simulink model "Commander_Stabilizer_QDrone_Follower"  (Simulink 9.1)
settings: Solver=ode1  StartTime=0.0  StopTime=inf  FixedStep=0.001  RelTol=1e-3  EnableMultiTasking=on
model workspace (MAT data in the model file):
  target_system : num (value not decoded)
InitFcn:
  | set_param(gcs, 'ZoomFactor','FitSystem')
undefined symbols (not defined in the file): HIL, qc_get_step_size
libraries: quarc_library x62, simulink x24, simulink_extras x5
(part 1 of 4)
settings Model: Creator=dmadill  LastModifiedBy=jpineros  SimulationMode=external  ExtModeTrigDuration=10000
settings SolverCC: PositivePriorityOrder=on
settings DataIOCC: LimitDataPoints=on
settings OptimizationCC: LifeSpan=auto
settings DebuggingCC: UnderspecifiedInitializationDetection=Simplified  MergeDetectMultiDrivingBlocksExec=error  SolverPrmCheckMsg=warning
settings HardwareCC: ProdBitPerLong=64  ProdBitPerPointer=64  ProdBitPerSizeT=64  ProdBitPerPtrDiffT=64  ProdLargestAtomicFloat=Float  ProdIntDivRoundTo=Zero  ProdEndianess=LittleEndian  ProdWordSize=64  ProdHWDeviceType=Intel->x86-64 (Linux 64)
settings RTWCC: SystemTargetFile=quarc_linux_x64.tlc  TemplateMakefile=quarc_linux_x64_tmf  Description=QUARC Linux x64 Target (QDrone)  BuildConfiguration=Faster Runs
settings STFCustomTargetCC: TargetLibSuffix=.a  ConcurrentExecutionCompliant=on  SystemTargetFile=quarc_linux_x64.tlc
settings GRTTargetCC: TargetLibSuffix=.a  TargetPreCompLibLocation=C:\PROGRA~3\QUARC\lib\2018a\LIA7F9~1\release  ParMdlRefBuildCompliant=off  CompOptLevelCompliant=off  MatFileLogging=off  CPPClassGenCompliant=off  UseToolchainInfoCompliant=off  ExtMode=on  ExtModeMexFile=quarc_comm  ExtModeMexArgs='-w -d /tmp -uri %u'
settings ConfigComp: CovHtmlReporting=off  CovSFcnEnable=off

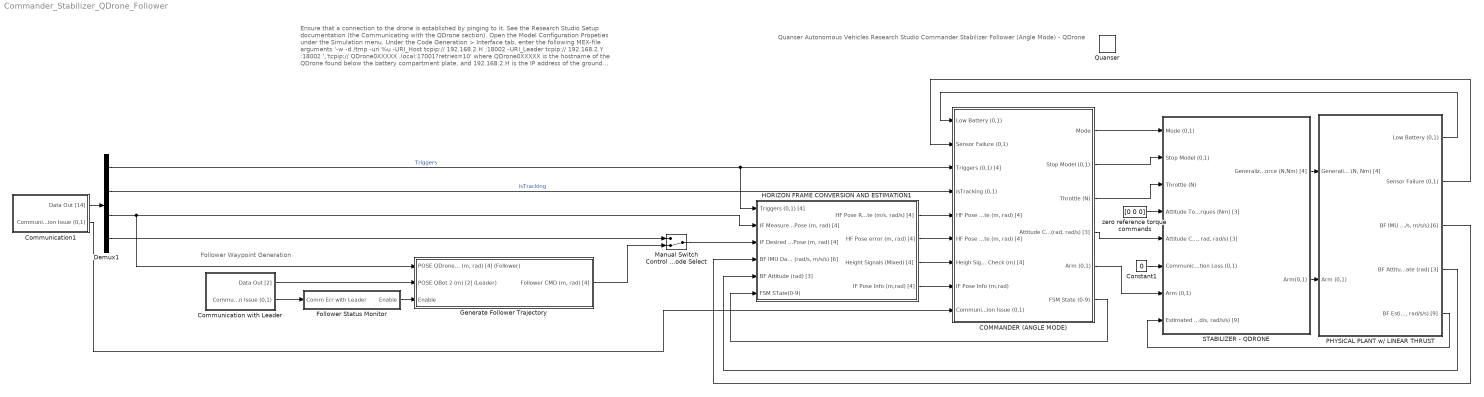
== system Commander_Stabilizer_QDrone_Follower ==
  note: Follower Waypoint Generation
  note: Quanser Autonomous Vehicles Research Studio
      | Commander Stabilizer Follower (Angle Mode) - QDrone
  note: Ensure that a connection to the drone is established by pinging to it. See the Research Studio Setup documentation (the Communicating with the QDrone section).
      | Open the Model Configuration Propeties under the Simulation menu.
      | Under the Code Generation > Interface tab, enter the following MEX-file arguments
      | '-w -d /tmp -uri %u -URI_Host tcpip:// 192.168.2.H :18002 -URI_Leader tcpip:// 192.168.2.Y :18002 ','tcpip:// QDrone0XXXXX .local:17001?retries=10'
      | where QDrone0XXXXX is the hostname of the QDrone found below the battery compartment plate, and 192.168.2.H is the IP address of the ground control station PC (should be 192.168.2.5 by default), 192.168.2.Y . is the IP address of the QBot2e which can be found on the custom Quanser PCB.
      |
      | Under the QUARC menu, click on Build .
      |
      | Ensure that the Mission Server Leader Follower model is running. If not, this model will stop immediately upon running. Click on Start under the QUARC menu.
      |
      | Ensure that the drone behaves as expected (see the steps in the Mission Server Leader Follower model)
      | This model will automatically stop when the QDrone lands.
  COMMANDER (ANGLE MODE) : Subsystem
  Communication with Leader : Subsystem
  Communication1 : Subsystem
  Constant1 : Constant  Value=0
  Demux1 : Demux  Outputs=[4 1 4 4]
  Follower Status Monitor : Subsystem
  Generate Follower Trajectory : Subsystem
  HORIZON FRAME CONVERSION AND ESTIMATION1 : Subsystem
  Manual Switch Control Mode Select : ManualSwitch  CurrentSetting=0
  PHYSICAL PLANT w/ LINEAR THRUST : Subsystem
  Quanser : quarc_library/Logos/Quanser
  STABILIZER - QDRONE : Subsystem
  zero reference torque commands : Constant  Value=[0 0 0]
  wires:
  Communication with Leader/1(Data Out [2]) -> Generate Follower Trajectory/2(POSE QBot 2 (m) [2] (Leader))
  Generate Follower Trajectory/1("Follower CMD (m, rad) [4]") -> Manual Switch Control Mode Select/2
  Follower Status Monitor/1(Enable) -> Generate Follower Trajectory/3(Enable)
  Communication with Leader/2(Communication Issue (0,1)) -> Follower Status Monitor/1(Comm Err with Leader)
  HORIZON FRAME CONVERSION AND ESTIMATION1/2("HF Pose error (m, rad) [4]") -> COMMANDER (ANGLE MODE)/6("HF Pose Error  Estimate (m, rad) [4]")
  HORIZON FRAME CONVERSION AND ESTIMATION1/1("HF Pose Rate  Estimate (m/s, rad/s) [4]") -> COMMANDER (ANGLE MODE)/5("HF Pose Rate  Estimate (m, rad) [4]")
  PHYSICAL PLANT w/ LINEAR THRUST/3("BF IMU Data (rad/s, m/s/s) [6]") -> HORIZON FRAME CONVERSION AND ESTIMATION1/4("BF IMU Data  (rad/s, m/s/s) [6]")
  COMMANDER (ANGLE MODE)/6(FSM State (0-9)) -> HORIZON FRAME CONVERSION AND ESTIMATION1/6(FSM STate(0-9))
  HORIZON FRAME CONVERSION AND ESTIMATION1/3(Height Signals (Mixed) [4]) -> COMMANDER (ANGLE MODE)/7(Heigh Signals Check (m) [4])
  Demux1/2 -> COMMANDER (ANGLE MODE)/4(isTracking (0,1))  "isTracking"
  Communication1/2(Communication Issue (0,1)) -> COMMANDER (ANGLE MODE)/9(Communication Issue (0,1))
  Demux1/3 -> Generate Follower Trajectory/1("POSE QDrone (m, rad) [4] (Follower)"), HORIZON FRAME CONVERSION AND ESTIMATION1/2("IF Measured Pose (m, rad) [4]")
  zero reference torque commands/1 -> STABILIZER - QDRONE/4(Attitude Torques (Nm) [3])
  COMMANDER (ANGLE MODE)/1(Mode) -> STABILIZER - QDRONE/1(Mode (0,1))
  COMMANDER (ANGLE MODE)/4("Attitude Commands (rad, rad/s) [3]") -> STABILIZER - QDRONE/5("Attitude Commands (rad, rad, rad/s) [3]")
  Demux1/1 -> COMMANDER (ANGLE MODE)/3(Triggers (0,1) [4]), HORIZON FRAME CONVERSION AND ESTIMATION1/1(Triggers (0,1) [4])  "Triggers"
  COMMANDER (ANGLE MODE)/3(Throttle (N)) -> STABILIZER - QDRONE/3(Throttle (N))
  Constant1/1 -> STABILIZER - QDRONE/6(Communication Loss (0,1))
  COMMANDER (ANGLE MODE)/5(Arm (0,1)) -> STABILIZER - QDRONE/7(Arm (0,1))
  Communication1/1(Data Out [14]) -> Demux1/1
  PHYSICAL PLANT w/ LINEAR THRUST/2(Sensor Failure (0,1)) -> COMMANDER (ANGLE MODE)/2(Sensor Failure (0,1))
  PHYSICAL PLANT w/ LINEAR THRUST/4(" BF Attitude Estimate (rad) [3]") -> HORIZON FRAME CONVERSION AND ESTIMATION1/5(BF Attitude (rad) [3])
  PHYSICAL PLANT w/ LINEAR THRUST/5("BF Estimated Attitude (rad, rad/s, rad/s/s) [9]") -> STABILIZER - QDRONE/8("Estimated Attitude (rad, rad/s, rad/s/s) [9]")
  STABILIZER - QDRONE/1(Generalized  Force (N,Nm) [4]) -> PHYSICAL PLANT w/ LINEAR THRUST/1("Generalized Force (N, Nm) [4]")
  STABILIZER - QDRONE/2(Arm(0,1)) -> PHYSICAL PLANT w/ LINEAR THRUST/2(Arm (0,1))
  COMMANDER (ANGLE MODE)/2(Stop Model (0,1)) -> STABILIZER - QDRONE/2(Stop Model (0,1))
  PHYSICAL PLANT w/ LINEAR THRUST/1(Low Battery (0,1)) -> COMMANDER (ANGLE MODE)/1(Low Battery (0,1))
  HORIZON FRAME CONVERSION AND ESTIMATION1/4(IF Pose Info (m,rad) [4]) -> COMMANDER (ANGLE MODE)/8(IF Pose Info (m,rad))
  Demux1/4 -> Manual Switch Control Mode Select/1
  Manual Switch Control Mode Select/1 -> HORIZON FRAME CONVERSION AND ESTIMATION1/3("IF Desired Pose (m, rad) [4]")

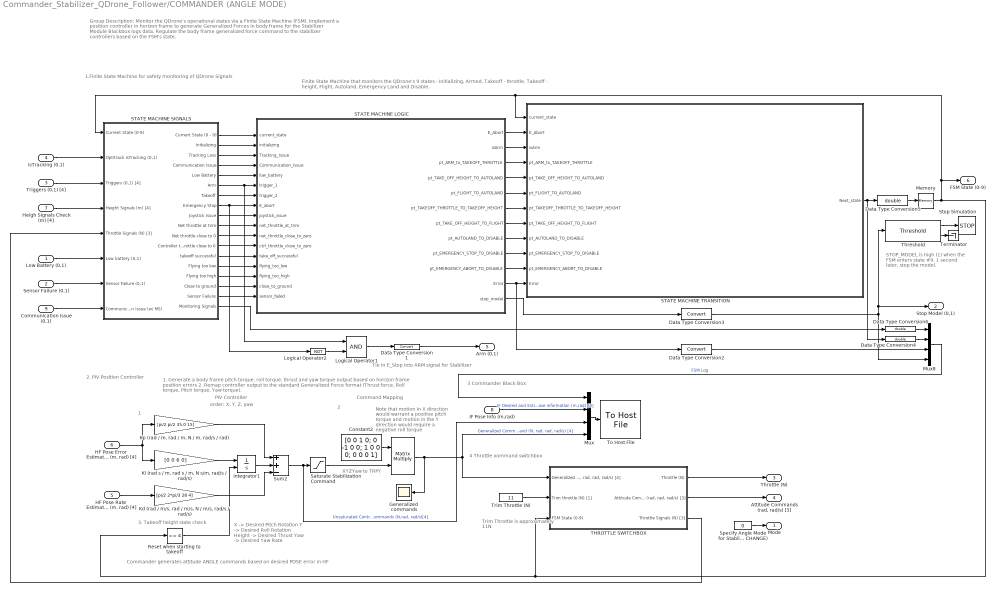
== system Commander_Stabilizer_QDrone_Follower/COMMANDER (ANGLE MODE) ==
  note: STOP_MODEL is high (1) when
      | the FSM enters state #9.
      | 1 second later, stop the model.
  note: Tie in E_Stop into ARM signal for Stabilizer
  note: Finite State Machine that monitors the QDrone's 9 states - Initializing, Armed, Takeoff - throttle, Takeoff - height, Flight, Autoland, Emergency Land and Disable.
  note: X -> Desired Pitch Rotation
      | Y -> Desired Roll Rotation
      | Height -> Desired Thrust
      | Yaw -> Desired Yaw Rate
  note: PIV Controller
  note: 2
  note: 1. Generate a body frame pitch torque, roll torque, thrust and yaw torque output based on horizon frame position errors
      | 2. Remap controller output to the standard Generalized Force format (Thrust force, Roll torque, Pitch torque, Yaw torque).
  note: order: X, Y, Z, yaw
  note: 3. Takeoff height state check
  note: 1
  note: XYZYaw to TRPY
  note: Command Mapping
  note: Note that motion in X direction would warrant a positive pitch torque
      | and motion in the Y direction would require a negative roll torque
  note: Trim Throttle is approximately 11N
  note: Group Description:
      |
      | Monitor the QDrone's operational states via a Finite State Machine (FSM).
      | Implement a position controller in horizon frame to generate Generalized Forces in body frame for the Stabilizer Module
      | Blackbox logs data.
      | Regulate the body frame generalized force command to the stabilizer controllers based on the FSM's state.
  note: 4 Throttle xommand switchbox
  note: 3 Commander Black Box
  note: Commander generates attitude ANGLE commands based on desired POSE error in HF
  note: 2. PIV Position Controller
  note: 1.Finite State Machine for safety monitoring of QDrone Signals
  Low Battery (0,1) : Inport
  Sensor Failure (0,1) : Inport  Port=2
  Triggers (0,1) [4] : Inport  Port=3
  isTracking (0,1) : Inport  Port=4
  "HF Pose Rate  Estimate (m, rad) [4]" : Inport  Port=5
  "HF Pose Error  Estimate (m, rad) [4]" : Inport  Port=6
  Heigh Signals Check (m) [4] : Inport  Port=7
  IF Pose Info (m,rad) : Inport  Port=8
  Communication Issue (0,1) : Inport  Port=9
  " " : Product  Multiplication=Matrix(*)
  Constant2 : Constant  Value=[0 0 1 0; 0 -1 0 0; 1 0 0 0; 0 0 0 1]
  Data Type Conversion1 : DataTypeConversion
  Data Type Conversion2 : DataTypeConversion
  Data Type Conversion3 : DataTypeConversion
  Data Type Conversion4 : DataTypeConversion  OutDataTypeStr=double
  Data Type Conversion5 : DataTypeConversion  OutDataTypeStr=double
  Data Type Conversion6 : DataTypeConversion  OutDataTypeStr=double
  "Generalized  commands " : Scope
  Integrator1 : Integrator  ExternalReset=rising  LimitOutput=on  UpperSaturationLimit=[0.26 0.33 15 0.05].*0.75  LowerSaturationLimit=[-0.26 -0.33 -15 -0.05].*0.75
  "Kd (rad / m/s, rad / m/s, N / m/s, rad/s / rad/s)" : Gain  Gain=[pi/2 2*pi/3 28 4]
  "Ki (rad s / m, rad s / m, N s/m, rad/s / rad/s)" : Gain  Gain=[0 0 6 0]
  "Kp (rad / m, rad / m, N / m, rad/s / rad)" : Gain  Gain=[pi/2 pi/2 35.0 15]
  Logical Operator1 : Logic  AllPortsSameDT=off  OutDataTypeStr=boolean
  Logical Operator2 : Logic  Operator=NOT  AllPortsSameDT=off  OutDataTypeStr=boolean
  Memory : Memory  InitialCondition=1
  Mux : Mux
  Mux8 : Mux  Inputs=[17 1 1 1]
  Reset when starting to takeoff : simulink/Logic and Bit Operations/Compare To Constant  relop===  const=4  OutDataTypeStr=boolean
  STATE MACHINE LOGIC : MATLAB Function  TreatAsAtomicUnit=on
  STATE MACHINE SIGNALS : Subsystem
  STATE MACHINE TRANSITION : MATLAB Function  TreatAsAtomicUnit=on
  Saturate Stabilization Command : Saturate  UpperLimit=[pi/4 pi/4 35 100*pi/180]  LowerLimit=[-pi/4 -pi/4 -35 -100*pi/180]
  Specify Angle Mode for Stabilizer (DO NOT CHANGE) : Constant  Value=0
  Stop Simulation : Stop
  Sum2 : Sum  Inputs=++-
  "THROTTLE SWITCHBOX " : Subsystem
  Terminator : Terminator
  Threshold : quarc_library/Discontinuities/Threshold  operator=>=  param_src=Specify via dialog  threshold=0.5  duration=1
      settings: SourceProductName=QUARC Targets
  To Host File : quarc_library/Sinks/To Host/To Host File  file_name=saved_data/%m/Commander_%{date}_%{time}.mat  variable_name=commander_data  decimation=1  sample_time=-1  file_format=MAT-file v.5  options=No header or footer  append=off  final_file_name=saved_data/Commander_Stabilizer_QDrone_Follower/Commander_20-Jan-2022_08-51-27.mat  bitrate=2000000
  "Trim Throttle (N) " : Constant  Value=11
  Mode : Outport
  Stop Model (0,1) : Outport  Port=2
  Throttle (N) : Outport  Port=3
  "Attitude Commands (rad, rad/s) [3]" : Outport  Port=4
  Arm (0,1) : Outport  Port=5
  FSM State (0-9) : Outport  Port=6
  wires:
  Heigh Signals Check (m) [4]/1 -> STATE MACHINE SIGNALS/4(Height Signals (m) [4])
  Triggers (0,1) [4]/1 -> STATE MACHINE SIGNALS/3(Triggers (0,1) [4])
  isTracking (0,1)/1 -> STATE MACHINE SIGNALS/2("Optitrack isTracking (0,1)  ")
  Communication Issue (0,1)/1 -> STATE MACHINE SIGNALS/8(Communication Issue (w/ MS))
  Sensor Failure (0,1)/1 -> STATE MACHINE SIGNALS/7(Sensor Failure (0,1))
  Low Battery (0,1)/1 -> STATE MACHINE SIGNALS/6(Low battery (0,1))
  STATE MACHINE LOGIC/11(Error) -> Data Type Conversion2/1, STATE MACHINE TRANSITION/12(Error)
  STATE MACHINE SIGNALS/17("  Sensor Failure") -> STATE MACHINE LOGIC/17(sensor_failed)
  STATE MACHINE LOGIC/8(pt_AUTOLAND_TO_DISABLE) -> STATE MACHINE TRANSITION/9(pt_AUTOLAND_TO_DISABLE)
  STATE MACHINE LOGIC/10(pt_EMERGENCY_ABORT_TO_DISABLE) -> STATE MACHINE TRANSITION/11(pt_EMERGENCY_ABORT_TO_DISABLE)
  Logical Operator2/1 -> Logical Operator1/2
  STATE MACHINE LOGIC/7(pt_TAKE_OFF_HEIGHT_TO_FLIGHT) -> STATE MACHINE TRANSITION/8(pt_TAKE_OFF_HEIGHT_TO_FLIGHT)
  STATE MACHINE SIGNALS/18(Monitoring Signals) -> Data Type Conversion6/1
  STATE MACHINE SIGNALS/6(Arm) -> STATE MACHINE LOGIC/6(trigger_1), Logical Operator1/1
  Logical Operator1/1 -> Data Type Conversion1/1
  Data Type Conversion2/1 -> Mux8/3
  Threshold/2 -> Terminator/1
  STATE MACHINE LOGIC/4(pt_TAKE_OFF_HEIGHT_TO_AUTOLAND) -> STATE MACHINE TRANSITION/5(pt_TAKE_OFF_HEIGHT_TO_AUTOLAND)
  Data Type Conversion3/1 -> Mux8/4, Threshold/1, Stop Model (0,1)/1
  STATE MACHINE LOGIC/2(isArm) -> STATE MACHINE TRANSITION/3(isArm)
  Data Type Conversion1/1 -> Arm (0,1)/1
  STATE MACHINE SIGNALS/2(Initializing) -> STATE MACHINE LOGIC/2(initializing)
  STATE MACHINE SIGNALS/3(Tracking Loss) -> STATE MACHINE LOGIC/3(Tracking_Issue)
  STATE MACHINE SIGNALS/10(Net throttle at trim) -> STATE MACHINE LOGIC/10(net_throttle_at_trim)
  STATE MACHINE SIGNALS/15(Flying too high) -> STATE MACHINE LOGIC/15(flying_too_high)
  STATE MACHINE SIGNALS/14(Flying too low) -> STATE MACHINE LOGIC/14(flying_too_low)
  STATE MACHINE SIGNALS/12(Controller throttle close to 0) -> STATE MACHINE LOGIC/12(ctrl_throttle_close_to_zero)
  Data Type Conversion4/1 -> Mux8/2
  STATE MACHINE SIGNALS/9("Joystick Issue ") -> STATE MACHINE LOGIC/9(joystick_issue)
  STATE MACHINE LOGIC/1(E_Abort) -> STATE MACHINE TRANSITION/2(E_Abort)
  STATE MACHINE LOGIC/5(pt_FLIGHT_TO_AUTOLAND) -> STATE MACHINE TRANSITION/6(pt_FLIGHT_TO_AUTOLAND)
  STATE MACHINE LOGIC/9(pt_EMERGENCY_STOP_TO_DISABLE) -> STATE MACHINE TRANSITION/10(pt_EMERGENCY_STOP_TO_DISABLE)
  STATE MACHINE SIGNALS/4(Communication Issue) -> STATE MACHINE LOGIC/4(Communication_Issue)
  STATE MACHINE TRANSITION/1(Next_state) -> Data Type Conversion4/1, Data Type Conversion5/1
  STATE MACHINE SIGNALS/7(Takeoff) -> STATE MACHINE LOGIC/7(trigger_2)
  STATE MACHINE SIGNALS/13(takeoff successful) -> STATE MACHINE LOGIC/13(take_off_successful)
  STATE MACHINE LOGIC/12(stop_model) -> Data Type Conversion3/1
  STATE MACHINE LOGIC/6(pt_TAKEOFF_THROTTLE_TO_TAKEOFF_HEIGHT) -> STATE MACHINE TRANSITION/7(pt_TAKEOFF_THROTTLE_TO_TAKEOFF_HEIGHT)
  STATE MACHINE SIGNALS/16(Close to ground) -> STATE MACHINE LOGIC/16(close_to_ground)
  STATE MACHINE SIGNALS/11(Net throttle close to 0) -> STATE MACHINE LOGIC/11(net_throttle_close_to_zero)
  Data Type Conversion6/1 -> Mux8/1
  STATE MACHINE SIGNALS/8(Emergency Stop) -> STATE MACHINE LOGIC/8(E_abort), Logical Operator2/1
  STATE MACHINE SIGNALS/5(Low Battery) -> STATE MACHINE LOGIC/5(low_battery)
  Data Type Conversion5/1 -> Memory/1
  STATE MACHINE LOGIC/3(pt_ARM_to_TAKEOFF_THROTTLE) -> STATE MACHINE TRANSITION/4(pt_ARM_to_TAKEOFF_THROTTLE)
  Threshold/1 -> Stop Simulation/1
  STATE MACHINE SIGNALS/1("Current State (0 - 9)  ") -> STATE MACHINE LOGIC/1(current_state)
  " "/1 -> Mux/4, "THROTTLE SWITCHBOX "/1("Generalized Command (N, rad, rad, rad/s) [4]"), "Generalized  commands "/1  "Generalized Command (N, rad, rad, rad/s) [4]"
  Reset when starting to takeoff/1 -> Integrator1/2
  Integrator1/1 -> Sum2/2
  "Kp (rad / m, rad / m, N / m, rad/s / rad)"/1 -> Sum2/1
  "HF Pose Rate  Estimate (m, rad) [4]"/1 -> "Kd (rad / m/s, rad / m/s, N / m/s, rad/s / rad/s)"/1
  Memory/1 -> STATE MACHINE SIGNALS/1(Current State (0-9)), STATE MACHINE TRANSITION/1(current_state), FSM State (0-9)/1, "THROTTLE SWITCHBOX "/3(FSM State (0-9)), Reset when starting to takeoff/1
  Constant2/1 -> " "/1
  Saturate Stabilization Command/1 -> " "/2
  "HF Pose Error  Estimate (m, rad) [4]"/1 -> "Kp (rad / m, rad / m, N / m, rad/s / rad)"/1, "Ki (rad s / m, rad s / m, N s/m, rad/s / rad/s)"/1
  "Kd (rad / m/s, rad / m/s, N / m/s, rad/s / rad/s)"/1 -> Sum2/3
  "Ki (rad s / m, rad s / m, N s/m, rad/s / rad/s)"/1 -> Integrator1/1
  Sum2/1 -> Saturate Stabilization Command/1, Mux/3  "Unsaturated Controller  Commands (N,rad, rad/s)[4]"
  "THROTTLE SWITCHBOX "/2("Attitude Command (rad, rad, rad/s) [3]") -> "Attitude Commands (rad, rad/s) [3]"/1
  IF Pose Info (m,rad)/1 -> Mux/2  "IF Desired and Estimated  pose information (m,rad) [8]"
  Mux/1 -> To Host File/1
  "THROTTLE SWITCHBOX "/3(Throttle Signals (N) [3]) -> STATE MACHINE SIGNALS/5(Throttle Signals (N) [3])
  "THROTTLE SWITCHBOX "/1(Throttle (N)) -> Throttle (N)/1
  "Trim Throttle (N) "/1 -> "THROTTLE SWITCHBOX "/2(Trim throttle (N) [1])
  Specify Angle Mode for Stabilizer (DO NOT CHANGE)/1 -> Mode/1
  Mux8/1 -> Mux/1  "FSM Log"

== system Commander_Stabilizer_QDrone_Follower/Communication with Leader ==
  note: Argument ( -URI_Leader ) is set at the MEX-file arguments found at Model Configuration Properties > Code Generation > Interface
      |
      | Format:
      | tcpip://192.168.2.Y:18002
      | where Y is the last digits of the Leader's IP address (use ipconfig in a command prompt to find it out).
  Constant : Constant
  Detect Communication Loss : Subsystem
  Memory : Memory  InheritSampleTime=on  LinearizeMemory=on  LinearizeAsDelay=on
  Model Argument : quarc_library/Sources/Signals/Model Argument  argument_name=URI_Leader  has_value=on  data_type_mode=Specify via dialog  data_type=char  max_length=80  default_value=0  variable_size=off
      settings: AttributesFormatString=(-%<argument_name>)  SourceProductName=QUARC Targets
  Select Timestamp received and send  back immediately (for calculating loopback time) : Selector  InputPortWidth=4  IndexOptions=Index vector (dialog)  Indices=[4]  OutputSizes=1
  Select the rest of the data : Selector  InputPortWidth=4  IndexOptions=Index vector (dialog)  Indices=[1:3]  OutputSizes=1
  Stream Client : quarc_library/Communications/Basic/Stream Client  uri_source=External input port  uri=tcpip://192.168.2.3:18669  apply_uri_to_all_configs=on  send_buffer_size=1460  receive_buffer_size=1460  byte_order=little endian (Intel - LSB first)  optimization=Minimum latency  send_options=Send most recent data  receive_options=Receive most recent data  default_value=zeros(1,4)  sample_time=qc_get_step_size  active=off  implementation=Use blocking I/O in a separate thread  send_fifo_size=1000  receive_fifo_size=1000  send_priority=0  receive_priority=0  send_dimensions=off  receive_dimensions=off  max_dimensions=-1  data_type=Inherited via back propagation  type_expr=BusObject
  String Display : quarc_library/Strings/String Display  alignment=center  display_mode=Single line  sample_time=-1  use_new=off
      settings: SourceProductName=QUARC Targets
  Terminator1 : Terminator
  Terminator2 : Terminator
  Data Out [2] : Outport
  Communication Issue (0,1) : Outport  Port=2
  wires:
  Memory/1 -> Stream Client/1
  Stream Client/3 -> Terminator1/1
  Constant/1 -> Stream Client/2
  Stream Client/5 -> Terminator2/1
  Select Timestamp received and send  back immediately (for calculating loopback time)/1 -> Memory/1
  Select the rest of the data/1 -> Data Out [2]/1
  Stream Client/1 -> Detect Communication Loss/1(State)
  Detect Communication Loss/1(Communication Issue) -> Communication Issue (0,1)/1
  Stream Client/2 -> Detect Communication Loss/2(Error)
  Stream Client/4 -> Detect Communication Loss/3(Data Out), Select the rest of the data/1, Select Timestamp received and send  back immediately (for calculating loopback time)/1
  Model Argument/1 -> Stream Client/3, String Display/1

== system Commander_Stabilizer_QDrone_Follower/Communication1 ==
  note: Argument (-URI_Host) is set at the MEX-file arguments found at Model Configuration Properties > Code Generation > Interface
      |
      | Format:
      | tcpip://192.168.2.H:18001
      | where H is the last digits of your ground station's IP address (use ipconfig in a command prompt to find it out).
  Constant : Constant
  Detect Communication Loss : Subsystem
  Memory : Memory  InheritSampleTime=on  LinearizeMemory=on  LinearizeAsDelay=on
  Model Argument : quarc_library/Sources/Signals/Model Argument  argument_name=URI_Host  has_value=on  data_type_mode=Specify via dialog  data_type=char  max_length=80  default_value=0  variable_size=off
      settings: AttributesFormatString=(-%<argument_name>)  SourceProductName=QUARC Targets
  Select Timestamp received and send  back immediately (for calculating loopback time) : Selector  InputPortWidth=14  IndexOptions=Index vector (dialog)  Indices=[14]  OutputSizes=1
  Select the rest of the data : Selector  InputPortWidth=14  IndexOptions=Index vector (dialog)  Indices=[1:13]  OutputSizes=1
  Stream Client : quarc_library/Communications/Basic/Stream Client  uri_source=External input port  uri=tcpip://192.168.2.3:18669  apply_uri_to_all_configs=on  send_buffer_size=1460  receive_buffer_size=1460  byte_order=little endian (Intel - LSB first)  optimization=Minimum latency  send_options=Send most recent data  receive_options=Receive most recent data  default_value=zeros(1,14)  sample_time=qc_get_step_size  active=off  implementation=Use blocking I/O in a separate thread  send_fifo_size=1000  receive_fifo_size=1000  send_priority=0  receive_priority=0  send_dimensions=off  receive_dimensions=off  max_dimensions=-1  data_type=Inherited via back propagation  type_expr=BusObject
  String Display : quarc_library/Strings/String Display  alignment=center  display_mode=Single line  sample_time=-1  use_new=off
      settings: SourceProductName=QUARC Targets
  Terminator1 : Terminator
  Terminator2 : Terminator
  Data Out [14] : Outport
  Communication Issue (0,1) : Outport  Port=2
  wires:
  Stream Client/5 -> Terminator2/1
  Model Argument/1 -> Stream Client/3, String Display/1
  Constant/1 -> Stream Client/2
  Stream Client/3 -> Terminator1/1
  Stream Client/4 -> Detect Communication Loss/3(Data Out), Select Timestamp received and send  back immediately (for calculating loopback time)/1, Select the rest of the data/1
  Memory/1 -> Stream Client/1
  Stream Client/1 -> Detect Communication Loss/1(State)
  Stream Client/2 -> Detect Communication Loss/2(Error)
  Detect Communication Loss/1(Communication Issue) -> Communication Issue (0,1)/1
  Select the rest of the data/1 -> Data Out [14]/1  "isTracking Triggers IF Measured Pose  IF Desired Pose"
  Select Timestamp received and send  back immediately (for calculating loopback time)/1 -> Memory/1

== system Commander_Stabilizer_QDrone_Follower/Follower Status Monitor ==
  note: Enable following only AFTER 1 second has passed
      | (to allow for sampling of Leader position) AND
      | no communication error with Leader.
  Comm Err with Leader : Inport
  AND : Logic  IconShape=distinctive  AllPortsSameDT=off  OutDataTypeStr=boolean
  Clock : Clock
  Compare To Constant : simulink/Logic and Bit Operations/Compare To Constant  relop=>=  const=1  OutDataTypeStr=boolean
  NOT : Logic  Operator=NOT  IconShape=distinctive  AllPortsSameDT=off  OutDataTypeStr=boolean
  Scope : Scope
  Scope1 : Scope
  Enable : Outport
  wires:
  Clock/1 -> Compare To Constant/1
  Compare To Constant/1 -> AND/1
  NOT/1 -> AND/2
  Comm Err with Leader/1 -> Scope1/1, NOT/1
  AND/1 -> Scope/1, Enable/1

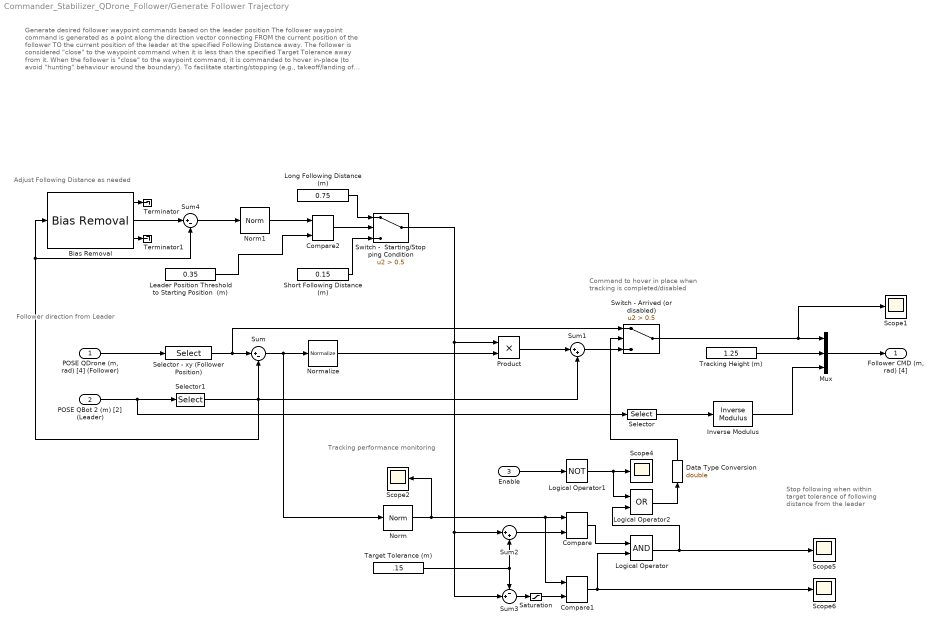
== system Commander_Stabilizer_QDrone_Follower/Generate Follower Trajectory ==
  note: Adjust Following Distance as needed
  note: Generate desired follower waypoint commands based on the leader position
      |
      | The follower waypoint command is generated as a point along the direction vector connecting FROM the current position of the follower TO the current position of the leader at the specified Following Distance away.
      |
      | The follower is considered "close" to the waypoint command when it is less than the specified Target Tolerance away from it.
      |
      | When the follower is "close" to the waypoint command, it is commanded to hover in-place (to avoid "hunting" behaviour around the boundary).
      |
      | To facilitate starting/stopping (e.g., takeoff/landing of the QDrone as follower), the Following Distance is adjusted (larger value for starting/stopping, smaller for normal tracking/following operation).
      |
      | Assumption: To identify starting/stopping condition, the Leader initial position at Follower model start is saved. Whenever the Leader returns to the initial position, it is assumed to be the stopping condition
      | (i.e., the Leader's starting and stopping positions are assumed to be the same). At that point, a larger Following Distance is used to keep the Follower stay clear of the Leader (to allow for collision free landing).
      |
      | There is an Enable signal override. If set to ZERO, the follower/tracking mode is turned off and the Follower is commanded to stay in its current position.
  note: Command to hover in place when
      | tracking is completed/disabled
  note: Stop following when
      | within target tolerance
      | of following distance from
      | the leader
  note: Tracking performance monitoring
  note: Follower direction from Leader
  "POSE QDrone (m, rad) [4] (Follower)" : Inport
  POSE QBot 2 (m) [2] (Leader) : Inport  Port=2
  Enable : Inport  Port=3
  Bias Removal : quarc_library/Discrete/Bias Removal  start_time=0  end_time=1  switch_id=0  sample_time=qc_get_step_size
      settings: SourceProductName=QUARC Targets
  Compare : quarc_library/Logic Operations/Compare  operator=<=  output_data_type=boolean
      settings: SourceProductName=QUARC Targets
  Compare1 : quarc_library/Logic Operations/Compare  operator=>=  output_data_type=boolean
      settings: SourceProductName=QUARC Targets
  Compare2 : quarc_library/Logic Operations/Compare  operator=<=  output_data_type=boolean
      settings: SourceProductName=QUARC Targets
  Data Type Conversion : DataTypeConversion  OutDataTypeStr=double
  Inverse Modulus : quarc_library/Discontinuities/Inverse Modulus  modulus=2*pi  output_derivative=off  output_revolutions=off  max_x=Inf  min_x=-Inf
  Leader Position Threshold to Starting Position  (m) : Constant  Value=0.35
  Logical Operator : Logic  AllPortsSameDT=off  OutDataTypeStr=boolean
  Logical Operator1 : Logic  Operator=NOT  Inputs=1  AllPortsSameDT=off  OutDataTypeStr=boolean
  Logical Operator2 : Logic  Operator=OR  AllPortsSameDT=off  OutDataTypeStr=boolean
  Long Following Distance (m) : Constant  Value=0.75
  Mux : Mux  Inputs=3
  Norm : quarc_library/Math Operations/Vectors/Norm
      settings: SourceProductName=QUARC Targets
  Norm1 : quarc_library/Math Operations/Vectors/Norm
      settings: SourceProductName=QUARC Targets
  Normalize : quarc_library/Math Operations/Vectors/Normalize
      settings: SourceProductName=QUARC Targets
  Product : Product
  Saturation : Saturate  UpperLimit=3  LowerLimit=0
  Scope{1..2,4..6} (5 alike) : Scope
  Selector : Selector  InputPortWidth=3  IndexOptions=Index vector (dialog)  Indices=[3]  OutputSizes=1
  Selector - xy (Follower Position) : Selector  InputPortWidth=4  IndexOptions=Index vector (dialog)  Indices=[1 2]  OutputSizes=1
  Selector1 : Selector  InputPortWidth=3  IndexOptions=Index vector (dialog)  Indices=[1 ,2]  OutputSizes=1
  Short Following Distance (m) : Constant  Value=0.15
  Sum : Sum  Inputs=|+-
  Sum1 : Sum  Inputs=|++
  Sum2 : Sum  Inputs=|++
  Sum3 : Sum  Inputs=-+|
  Sum4 : Sum  Inputs=|+-
  Switch -  Starting/Stopping Condition : Switch  Criteria=u2 > Threshold  Threshold=0.5
  Switch - Arrived (or disabled) : Switch  Criteria=u2 > Threshold  Threshold=0.5
  Target Tolerance (m) : Constant  Value=.15
  Terminator : Terminator
  Terminator1 : Terminator
  Tracking Height (m) : Constant  Value=1.25
  "Follower CMD (m, rad) [4]" : Outport
  wires:
  "POSE QDrone (m, rad) [4] (Follower)"/1 -> Selector - xy (Follower Position)/1
  Product/1 -> Sum1/1
  Normalize/1 -> Product/2
  Tracking Height (m)/1 -> Mux/2
  POSE QBot 2 (m) [2] (Leader)/1 -> Selector1/1, Selector/1
  Mux/1 -> "Follower CMD (m, rad) [4]"/1
  Sum2/1 -> Compare/2
  Target Tolerance (m)/1 -> Sum2/2, Sum3/1
  Norm/1 -> Compare1/1, Compare/1, Scope2/1
  Enable/1 -> Logical Operator1/1
  Logical Operator1/1 -> Scope4/1, Logical Operator2/1
  Logical Operator/1 -> Logical Operator2/2, Scope5/1
  Bias Removal/2 -> Sum4/1
  Sum4/1 -> Norm1/1
  Norm1/1 -> Compare2/1
  Compare2/1 -> Switch -  Starting/Stopping Condition/2
  Long Following Distance (m)/1 -> Switch -  Starting/Stopping Condition/1
  Switch -  Starting/Stopping Condition/1 -> Product/1, Sum2/1, Sum3/2
  Short Following Distance (m)/1 -> Switch -  Starting/Stopping Condition/3
  Leader Position Threshold to Starting Position  (m)/1 -> Compare2/2
  Bias Removal/1 -> Terminator/1
  Bias Removal/3 -> Terminator1/1
  Sum/1 -> Norm/1, Normalize/1
  Sum1/1 -> Switch - Arrived (or disabled)/3
  Compare/1 -> Logical Operator/1
  Compare1/1 -> Logical Operator/2, Scope6/1
  Sum3/1 -> Saturation/1
  Saturation/1 -> Compare1/2
  Selector - xy (Follower Position)/1 -> Sum/1, Switch - Arrived (or disabled)/1
  Data Type Conversion/1 -> Switch - Arrived (or disabled)/2
  Logical Operator2/1 -> Data Type Conversion/1
  Switch - Arrived (or disabled)/1 -> Mux/1, Scope1/1
  Selector1/1 -> Sum4/2, Bias Removal/1, Sum1/2, Sum/2
  Selector/1 -> Inverse Modulus/1
  Inverse Modulus/1 -> Mux/3

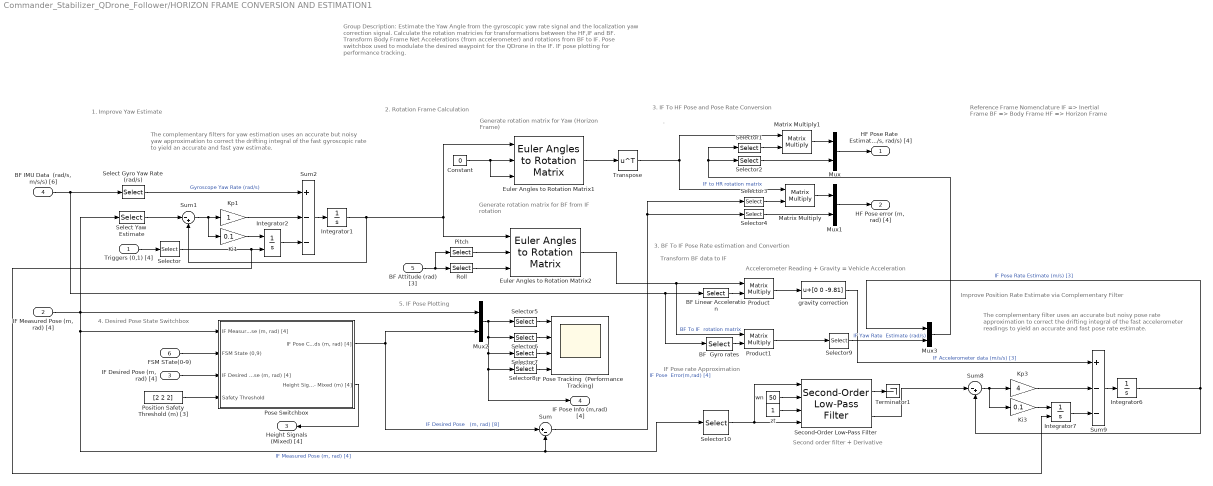
== system Commander_Stabilizer_QDrone_Follower/HORIZON FRAME CONVERSION AND ESTIMATION1 ==
  note: 3. IF To HF Pose and Pose Rate Conversion
  note: IF Pose rate Approximation
  note: Transform BF data to IF
  note: 3. BF To IF Pose Rate estimation and Convertion
  note: 2. Rotation Frame Calculation
  note: .
  note: Reference Frame Nomenclature
      | IF => Inertial Frame
      | BF => Body Frame
      | HF => Horizon Frame
  note: Group Description:
      |
      | Estimate the Yaw Angle from the gyroscopic yaw rate signal and the localization yaw correction signal.
      | Calculate the rotation matricies for transformations between the HF,IF and BF.
      | Transform Body Frame Net Accelerations (from accelerometer) and rotations from BF to IF.
      | Pose switchbox used to modulate the desired waypoint for the QDrone in the IF.
      | IF pose plotting for performance tracking.
  note: 4. Desired Pose State Switchbox
  note: 5. IF Pose Plotting
  note: 1. Improve Yaw Estimate
  note: The complementary filters for yaw estimation uses an accurate but noisy yaw approximation to correct the drifting integral of the fast gyroscopic rate to yield an accurate and fast yaw estimate.
  note: Generate rotation matrix for Yaw
      | (Horizon Frame)
  note: Generate rotation matrix
      | for BF from IF rotation
  note: Accelerometer Reading + Gravity = Vehicle Acceleration
  note: The complementary filter uses an accurate but noisy pose rate approximation to correct the drifting integral of the fast accelerometer readings to yield an accurate and fast pose rate estimate.
  note: Second order filter + Derivative
  note: Improve Position Rate Estimate via Complementary Filter
  Triggers (0,1) [4] : Inport
  "IF Measured Pose (m, rad) [4]" : Inport  Port=2
  "IF Desired Pose (m, rad) [4]" : Inport  Port=3
  "BF IMU Data  (rad/s, m/s/s) [6]" : Inport  Port=4
  BF Attitude (rad) [3] : Inport  Port=5
  FSM STate(0-9) : Inport  Port=6
  BF  Gyro rates : Selector  InputPortWidth=6  IndexOptions=Index vector (dialog)  Indices=[1:3]  OutputSizes=1
  BF Linear Acceleration : Selector  InputPortWidth=6  IndexOptions=Index vector (dialog)  Indices=[4:6]  OutputSizes=1
  Constant : Constant  Value=0
  Euler Angles to Rotation Matrix1 : quarc_library/Math Operations/Matrices/Euler Angles to Rotation Matrix  menu_order=Relative Z-Y-X
      settings: SourceProductName=QUARC Targets
  Euler Angles to Rotation Matrix2 : quarc_library/Math Operations/Matrices/Euler Angles to Rotation Matrix  menu_order=Relative Z-Y-X
      settings: SourceProductName=QUARC Targets
  IF Pose Tracking  (Performance Tracking) : Scope  NumInputPorts=4
  Integrator1 : Integrator
  Integrator2 : Integrator  ExternalReset=rising
  Integrator6 : Integrator
  Integrator7 : Integrator  ExternalReset=rising
  Ki1 : Gain  Gain=0.1
  Ki3 : Gain  Gain=0.1
  Kp1 : Gain
  Kp3 : Gain  Gain=4
  Matrix Multiply : Product  Multiplication=Matrix(*)
  Matrix Multiply1 : Product  Multiplication=Matrix(*)
  Mux{,1..3} (4 alike) : Mux  Inputs=2
  Pitch : Selector  InputPortWidth=3  IndexOptions=Index vector (dialog)  Indices=[2]  OutputSizes=1
  Pose Switchbox : Subsystem
  Position Safety Threshold (m) [3] : Constant  Value=[2 2 2]
  Product : Product  Multiplication=Matrix(*)
  Product1 : Product  Multiplication=Matrix(*)
  Roll : Selector  InputPortWidth=3  IndexOptions=Index vector (dialog)  Indices=[1]  OutputSizes=1
  Second-Order Low-Pass Filter : quarc_library/Continuous/Second-Order Low-Pass Filter  params_source=External (input ports)  input_width=1  input_zeta=1  input_init=0
  Select Gyro Yaw Rate (rad/s) : Selector  InputPortWidth=6  IndexOptions=Index vector (dialog)  Indices=[3]  OutputSizes=1
  Select Yaw Estimate : Selector  InputPortWidth=4  IndexOptions=Index vector (dialog)  Indices=4  OutputSizes=1
  Selector : Selector  InputPortWidth=4  IndexOptions=Index vector (dialog)  Indices=[2]  OutputSizes=1
  Selector1 : Selector  InputPortWidth=4  IndexOptions=Index vector (dialog)  Indices=[1:3]  OutputSizes=1
  Selector10 : Selector  InputPortWidth=4  IndexOptions=Index vector (dialog)  Indices=[1:3]  OutputSizes=1
  Selector2 : Selector  InputPortWidth=4  IndexOptions=Index vector (dialog)  Indices=[4]  OutputSizes=1
  Selector3 : Selector  InputPortWidth=4  IndexOptions=Index vector (dialog)  Indices=[1:3]  OutputSizes=1
  Selector4 : Selector  InputPortWidth=4  IndexOptions=Index vector (dialog)  Indices=[4]  OutputSizes=1
  Selector5 : Selector  InputPortWidth=8  IndexOptions=Index vector (dialog)  Indices=[1 5]  OutputSizes=1
  Selector6 : Selector  InputPortWidth=8  IndexOptions=Index vector (dialog)  Indices=[2 6]  OutputSizes=1
  Selector7 : Selector  InputPortWidth=8  IndexOptions=Index vector (dialog)  Indices=[3 7]  OutputSizes=1
  Selector8 : Selector  InputPortWidth=8  IndexOptions=Index vector (dialog)  Indices=[4 8]  OutputSizes=1
  Selector9 : Selector  InputPortWidth=3  IndexOptions=Index vector (dialog)  Indices=[3]  OutputSizes=1
  Sum : Sum  Inputs=|+-
  Sum1 : Sum  Inputs=|-+
  Sum2 : Sum  Inputs=+--
  Sum8 : Sum  Inputs=|-+
  Sum9 : Sum  Inputs=+--
  Terminator1 : Terminator
  Transpose : Math  Operator=transpose  SaturateOnIntegerOverflow=on
  gravity correction : Bias  Bias=[0 0 -9.81]
  wn : Constant  Value=50
  zt : Constant
  "HF Pose Rate  Estimate (m/s, rad/s) [4]" : Outport
  "HF Pose error (m, rad) [4]" : Outport  Port=2
  Height Signals (Mixed) [4] : Outport  Port=3
  IF Pose Info (m,rad) [4] : Outport  Port=4
  wires:
  Selector5/1 -> IF Pose Tracking  (Performance Tracking)/1
  Selector7/1 -> IF Pose Tracking  (Performance Tracking)/3
  Mux2/1 -> Selector6/1, Selector7/1, Selector8/1, IF Pose Info (m,rad) [4]/1, Selector5/1
  Selector6/1 -> IF Pose Tracking  (Performance Tracking)/2
  Selector8/1 -> IF Pose Tracking  (Performance Tracking)/4
  Selector4/1 -> Mux1/2
  Matrix Multiply/1 -> Mux1/1
  Selector3/1 -> Matrix Multiply/2
  Pose Switchbox/2(Height Signals - Mixed (m) [4]) -> Height Signals (Mixed) [4]/1
  Mux/1 -> "HF Pose Rate  Estimate (m/s, rad/s) [4]"/1
  Selector2/1 -> Mux/2
  Selector1/1 -> Matrix Multiply1/2
  Matrix Multiply1/1 -> Mux/1
  Transpose/1 -> Matrix Multiply/1, Matrix Multiply1/1  "IF to HR rotation matrix"
  Mux3/1 -> Selector1/1, Selector2/1
  Mux1/1 -> "HF Pose error (m, rad) [4]"/1
  Sum/1 -> Selector3/1, Selector4/1  "IF Pose  Error(m,rad) [4]"
  FSM STate(0-9)/1 -> Pose Switchbox/2(FSM State (0,9))
  Position Safety Threshold (m) [3]/1 -> Pose Switchbox/4(Safety Threshold)
  "BF IMU Data  (rad/s, m/s/s) [6]"/1 -> Select Gyro Yaw Rate (rad/s)/1, BF Linear Acceleration/1, BF  Gyro rates/1
  Select Gyro Yaw Rate (rad/s)/1 -> Sum2/1  "Gyroscope Yaw Rate (rad/s)"
  Triggers (0,1) [4]/1 -> Selector/1
  BF Attitude (rad) [3]/1 -> Pitch/1, Roll/1
  "IF Desired Pose (m, rad) [4]"/1 -> Pose Switchbox/3("IF Desired Pose (m, rad) [4]")
  BF Linear Acceleration/1 -> Product/2
  BF  Gyro rates/1 -> Product1/2
  Integrator2/1 -> Sum2/3
  Select Yaw Estimate/1 -> Sum1/1
  Sum1/1 -> Ki1/1, Kp1/1
  Kp1/1 -> Sum2/2
  Sum2/1 -> Integrator1/1
  Ki1/1 -> Integrator2/1
  Roll/1 -> Euler Angles to Rotation Matrix2/3
  Pitch/1 -> Euler Angles to Rotation Matrix2/2
  Constant/1 -> Euler Angles to Rotation Matrix1/3, Euler Angles to Rotation Matrix1/2
  Integrator1/1 -> Sum1/2, Euler Angles to Rotation Matrix2/1, Euler Angles to Rotation Matrix1/1
  Euler Angles to Rotation Matrix1/1 -> Transpose/1
  Product1/1 -> Selector9/1
  Product/1 -> gravity correction/1
  Euler Angles to Rotation Matrix2/1 -> Product/1, Product1/1  "BF To IF  rotation matrix"
  Selector10/1 -> Second-Order Low-Pass Filter/1, Second-Order Low-Pass Filter/4
  Kp3/1 -> Sum9/2
  gravity correction/1 -> Sum9/1  "IF Accelerometer data (m/s/s) [3]"
  Second-Order Low-Pass Filter/2 -> Sum8/1
  Second-Order Low-Pass Filter/1 -> Terminator1/1
  zt/1 -> Second-Order Low-Pass Filter/3
  Ki3/1 -> Integrator7/1
  Sum8/1 -> Ki3/1, Kp3/1
  Integrator6/1 -> Sum8/2, Mux3/1  "IF Pose Rate Estimate (m/s) [3]"
  Sum9/1 -> Integrator6/1
  wn/1 -> Second-Order Low-Pass Filter/2
  Integrator7/1 -> Sum9/3
  Selector/1 -> Integrator2/2, Integrator7/2
  Selector9/1 -> Mux3/2  "IF Yaw Rate  Estimate (rad/s)"
  "IF Measured Pose (m, rad) [4]"/1 -> Select Yaw Estimate/1, Sum/2, Selector10/1, Pose Switchbox/1("IF Measured Pose (m, rad) [4]"), Mux2/1  "IF Measured Pose (m, rad) [4]"
  Pose Switchbox/1("IF Pose Commands (m, rad) [4]") -> Mux2/2, Sum/1  "IF Desired Pose   (m, rad) [8]"
